simulink model "RRR_BS"  (R2022a)
settings: Solver=VariableStepAuto  StartTime=0.0  StopTime=500  RelTol=1e-6
undefined symbols (not defined in the file): DiscIntNeverNeededParam, dq0, Ks_BS, Levenberg, m1, m2, m3, Marquardt, p0, param, q0, r0, r1, r2, rel_err, slow
libraries: robotmaniplib x2, simulink x1
settings Model: PauseTimes=0.14  Creator=Mathew  LastModifiedBy=Marco
settings SolverCC: ZeroCrossControl=DisableAll  ODENIntegrationMethod=ode1be
settings DebuggingCC: AlgebraicLoopMsg=none  UnconnectedInputMsg=warning  UnconnectedOutputMsg=warning  UnconnectedLineMsg=warning  SFMachineParentedDataDiag=warning
settings SFSimCC: CustomCodeUndefinedFunction=UseInterfaceOnly
settings RTWCC: DLArmComputeVersion=19.05

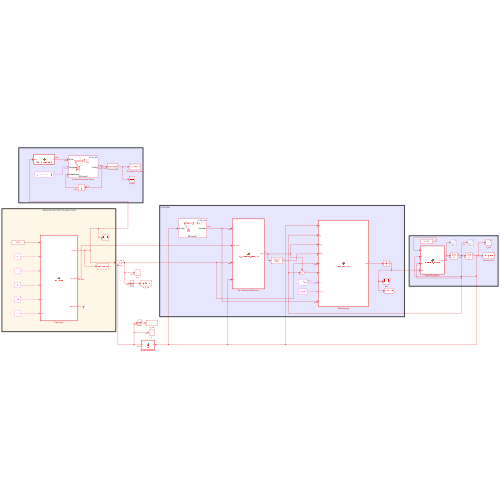
[thumbnail: Simulink's stored preview of the top-level diagram]
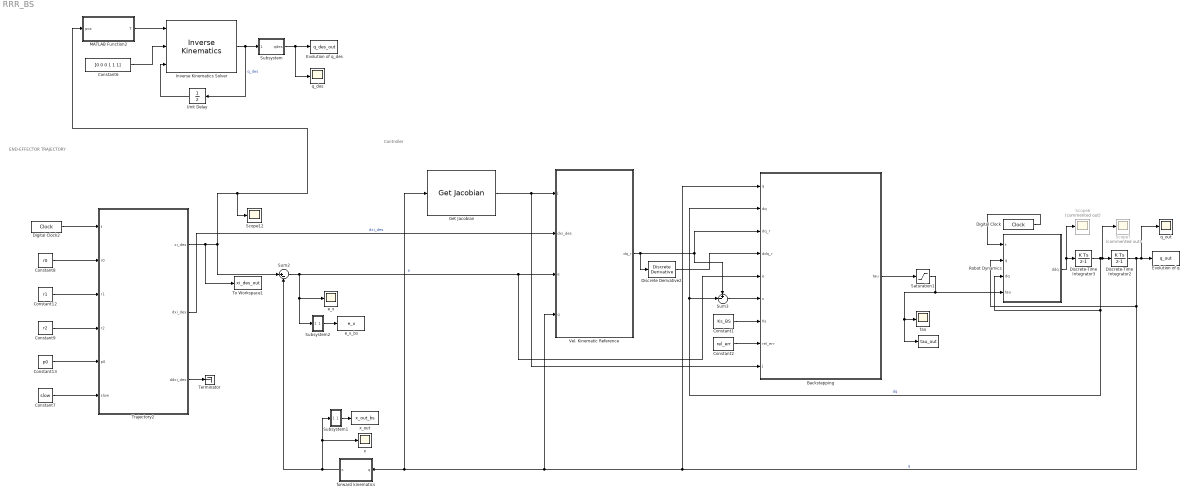
== system RRR_BS ==
  note: Controller
  note: END-EFFECTOR TRAJECTORY
  "         " : ToWorkspace  VariableName=tau_out  SaveFormat=Timeseries  SampleTime=-1
  Backstepping : MATLAB Function  TreatAsAtomicUnit=on
  Constant1 : Constant  Value=Ks_BS
  Constant12 : Constant  Value=r1
  Constant13 : Constant  Value=p0
  Constant2 : Constant  Value=rel_err
  Constant6 : Constant  Value=[0 0 0 1 1 1]
  Constant7 : Constant  Value=slow
  Constant8 : Constant  Value=r0
  Constant9 : Constant  Value=r2
  Digital Clock : DigitalClock  SampleTime=0.01
  Digital Clock2 : DigitalClock  SampleTime=0.01
  Discrete Derivative2 : simulink/Discrete/Discrete Derivative  gainval=1.0  ICPrevScaledInput=ddq0  OutMin=[]  OutMax=[]  OutDataType=fixdt(1, 16)  OutScaling=2^-10  DoSatur=off
  Discrete-Time Integrator2 : DiscreteIntegrator  InitialCondition=q0  SampleTime=-1  ICPrevOutput=DiscIntNeverNeededParam  ICPrevScaledInput=DiscIntNeverNeededParam
  Discrete-Time Integrator3 : DiscreteIntegrator  InitialCondition=dq0  SampleTime=-1  ICPrevOutput=DiscIntNeverNeededParam  ICPrevScaledInput=DiscIntNeverNeededParam
  Evolution of q : ToWorkspace  VariableName=q_out  SaveFormat=Timeseries  SampleTime=-1
  Evolution of q_des : ToWorkspace  VariableName=q_des_out  SaveFormat=Timeseries  SampleTime=-1
  Get Jacobian : robotmaniplib/Get Jacobian  RigidBodyTree=ur10e_bis  EndEffector=body3  SimulateUsing=Interpreted execution
      settings: SourceProductBaseCode=RO
  Inverse Kinematics Solver : robotmaniplib/Inverse Kinematics  RigidBodyTree=ur10e_bis  EndEffector=body3  ShowInfo=off  SolverName=Levenberg-Marquardt  EnforceJointLimits=on  MaxIterations=1500  MaxTime=10  GradientTolerance=1e-7  SolutionTolerance=1e-5  StepTolerance=1e-14  ErrorChangeTolerance=1e-8  UseErrorDamping=on  DampingBias=0.0025  SimulateUsing=Interpreted execution
  MATLAB Function2 : MATLAB Function  TreatAsAtomicUnit=on
  Robot Dynamics : MATLAB Function  TreatAsAtomicUnit=on
  Saturation1 : Saturate  UpperLimit=100  LowerLimit=-100
  Scope12 : Scope
  Scope6 : Scope  Commented=on
  Scope7 : Scope  Commented=on
  Subsystem : Subsystem
  Subsystem1 : Subsystem
  Subsystem2 : Subsystem
  Sum2 : Sum  Inputs=|+-
  Sum3 : Sum  Inputs=+-|
  Terminator : Terminator
  To Workspace1 : ToWorkspace  VariableName=xi_des_out  SaveFormat=Timeseries  SampleTime=-1
  Trajectory2 : MATLAB Function  TreatAsAtomicUnit=on
  Unit Delay : UnitDelay  SampleTime=-1  HasFrameUpgradeWarning=on
  "Vel. Kinematic Reference " : MATLAB Function  TreatAsAtomicUnit=on
  e_x : Scope
  e_x_bs : ToWorkspace  VariableName=e_x  SaveFormat=Timeseries  SampleTime=-1
  forward kinematics : MATLAB Function  TreatAsAtomicUnit=on
  q_des : Scope
  q_out : Scope
  tau : Scope
  x : Scope
  x_out : ToWorkspace  VariableName=x_out_bs  SaveFormat=Timeseries  SampleTime=-1
  wires:
  Backstepping/1(tau) -> Saturation1/1
  Saturation1/1 -> "         "/1, tau/1, Robot Dynamics/4(tau)
  Discrete-Time Integrator3/1 -> Backstepping/2(dq), Sum3/2, Robot Dynamics/3(dq), Scope7/1, Discrete-Time Integrator2/1  "dq"
  Discrete-Time Integrator2/1 -> Get Jacobian/1, forward kinematics/1(q), "Vel. Kinematic Reference "/4(q), Backstepping/1(q), Robot Dynamics/2(q), Evolution of q/1, q_out/1  "q"
  Robot Dynamics/1(ddq) -> Scope6/1, Discrete-Time Integrator3/1
  Inverse Kinematics Solver/1 -> Subsystem/1(q_des), Unit Delay/1  "q_des"
  Subsystem/1(qdes) -> Evolution of q_des/1, q_des/1
  Digital Clock/1 -> Robot Dynamics/1(t)
  Trajectory2/1(xi_des) -> MATLAB Function2/1(pos), Scope12/1, Sum2/1, To Workspace1/1
  Constant13/1 -> Trajectory2/5(p0)
  Constant7/1 -> Trajectory2/6(slow)
  Constant9/1 -> Trajectory2/4(r2)
  Constant12/1 -> Trajectory2/3(r1)
  Constant6/1 -> Inverse Kinematics Solver/2
  MATLAB Function2/1(T) -> Inverse Kinematics Solver/1
  Unit Delay/1 -> Inverse Kinematics Solver/3
  Digital Clock2/1 -> Trajectory2/1(t)
  Constant8/1 -> Trajectory2/2(r0)
  Constant1/1 -> Backstepping/7(Ks)
  Constant2/1 -> Backstepping/8(rel_err)
  "Vel. Kinematic Reference "/1(dq_r) -> Sum3/1, Backstepping/3(dq_r), Discrete Derivative2/1
  Discrete Derivative2/1 -> Backstepping/4(ddq_r)
  Sum3/1 -> Backstepping/6(s)
  Sum2/1 -> Backstepping/5(e), "Vel. Kinematic Reference "/3(e), Subsystem2/1(q_des), e_x/1  "e"
  Trajectory2/2(dxi_des) -> "Vel. Kinematic Reference "/2(dxi_des)  "dxi_des"
  Get Jacobian/1 -> Backstepping/9(J), "Vel. Kinematic Reference "/1(J)
  forward kinematics/1(x) -> Subsystem1/1(q_des), x/1, Sum2/2
  Trajectory2/3(ddxi_des) -> Terminator/1
  Subsystem1/1(qdes) -> x_out/1
  Subsystem2/1(qdes) -> e_x_bs/1

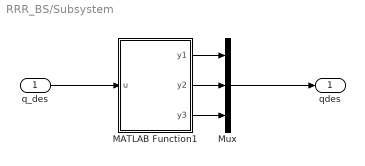
== system RRR_BS/Subsystem ==
  q_des : Inport
  MATLAB Function1 : MATLAB Function  TreatAsAtomicUnit=on
  Mux : Mux  Inputs=3
  qdes : Outport
  wires:
  MATLAB Function1/3(y3) -> Mux/3
  MATLAB Function1/2(y2) -> Mux/2
  q_des/1 -> MATLAB Function1/1(u)
  Mux/1 -> qdes/1
  MATLAB Function1/1(y1) -> Mux/1

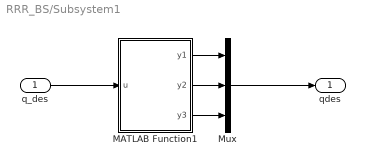
== system RRR_BS/Subsystem1 ==
  q_des : Inport
  MATLAB Function1 : MATLAB Function  TreatAsAtomicUnit=on
  Mux : Mux  Inputs=3
  qdes : Outport
  wires:
  MATLAB Function1/1(y1) -> Mux/1
  Mux/1 -> qdes/1
  q_des/1 -> MATLAB Function1/1(u)
  MATLAB Function1/2(y2) -> Mux/2
  MATLAB Function1/3(y3) -> Mux/3

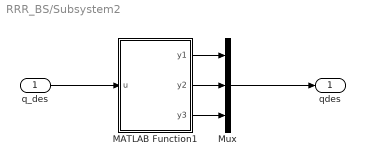
== system RRR_BS/Subsystem2 ==
  q_des : Inport
  MATLAB Function1 : MATLAB Function  TreatAsAtomicUnit=on
  Mux : Mux  Inputs=3
  qdes : Outport
  wires:
  MATLAB Function1/3(y3) -> Mux/3
  MATLAB Function1/2(y2) -> Mux/2
  q_des/1 -> MATLAB Function1/1(u)
  Mux/1 -> qdes/1
  MATLAB Function1/1(y1) -> Mux/1

== matlab function RRR_BS/Robot Dynamics ==
  data: t input; q input; dq input; tau input; ddq output; m1 parameter; m2 parameter; m3 parameter; param parameter
function ddq = inverse_dynamics(t, q, dq, tau,m1, m2, m3, param)
   
    g = 9.81;
    
    if t > 50
        m2=m2+1;
    end

    % Get dynamic matrices
    M = B_3r(param,m1,m2,m3,q);
    C = C_3r(param,m1,m2,m3,q,dq);
    G = G_3r(g,param,m1,m2,m3,q);
    
    ddq = pinv(M)*(tau - C*dq - G);

end

== matlab function RRR_BS/forward kinematics ==
  data: q input; x output; param parameter
function x = FK(q,param)
    T = eye(4);
    x = [0;0;0];

    T = FK_3r(param,q);

    x = T(1:3,4);

end

== matlab function RRR_BS/Subsystem1/MATLAB Function1 ==
  data: u input; y1 output; y2 output; y3 output
function [y1,y2,y3] = fcn(u)

y1 = squeeze(u(1));
y2 = squeeze(u(2));
y3 = squeeze(u(3));

== matlab function RRR_BS/Subsystem2/MATLAB Function1 ==
  data: u input; y1 output; y2 output; y3 output
function [y1,y2,y3] = fcn(u)

y1 = squeeze(u(1));
y2 = squeeze(u(2));
y3 = squeeze(u(3));

== matlab function RRR_BS/Vel. Kinematic Reference  ==
  data: J input; dxi_des input; dq_r output; e input; q input; Lambda_BS parameter
function dq_r = vel_kinematic_reference(J, dxi_des, e, q, Lambda_BS)

    % Computing jacobian
    J = J(4:6,1:3);
    
    dq_r = pinv(J) * (dxi_des + Lambda_BS*e);

end

== matlab function RRR_BS/Subsystem/MATLAB Function1 ==
  data: u input; y1 output; y2 output; y3 output
function [y1,y2,y3] = fcn(u)

y1 = squeeze(u(1));
y2 = squeeze(u(2));
y3 = squeeze(u(3));

== matlab function RRR_BS/Backstepping ==
  data: q input; dq input; dq_r input; tau output; ddq_r input; e input; s input; Ks input; rel_err input; m1 parameter; m2 parameter; m3 parameter; param parameter; J input
function tau = backstepping(q, dq, dq_r, ddq_r, e, s, Ks, rel_err,m1, m2, m3, param, J)

    J=J(4:6,1:3);

    g = 9.81;
    
    % Get dynamic matrices
    M = B_3r(param,m1,m2,m3,q);
    C = C_3r(param,m1,m2,m3,q,dq);
    G = G_3r(g,param,m1,m2,m3,q);
    
    % Adding uncertainty
    M = M.*(1 + rel_err);
    C = C.*(1 + rel_err);
    G = G.*(1 + rel_err);
    
    
    % Control law
    tau = M*ddq_r + C*dq_r + G + Ks*s + J.'*e;


end

== matlab function RRR_BS/Trajectory2 ==
  data: t input; r0 input; xi_des output; r1 input; r2 input; p0 input; slow input; dxi_des output; ddxi_des output
function [xi_des, dxi_des, ddxi_des] = trajectory(t,r0,r1,r2,p0,slow)

    k=slow;
    
    xi_des =   [r0*sin(t/(2*k))       ; r1*sin(t/k)     ; r2*cos(t/k)     ] + p0;
    dxi_des =  [r0/2/k*cos(t/(2*k))   ; r1/k*cos(t/k)   ; -r2/k*sin(t/k)  ];
    ddxi_des = [-r0/4/k/k*sin(t/(2*k)); -r1/k/k*sin(t/k); -r2/k/k*cos(t/k)];

end

== matlab function RRR_BS/MATLAB Function2 ==
  data: pos input; T output
function T = homogeneus_transf(pos)
    
    T=eye(4);
    
    T = [  eye(3),     [pos(1);pos(2);pos(3) ];
         0 0 0              1           ]; 

end
